simulink model "Simulink_Model_For_MAE_171a_Control_Lab"  (R2024b)
settings: Solver=VariableStepAuto  StartTime=0.0  StopTime=10.0  RelTol=1e-3
values from neighbouring files (symbols this model uses):
  den = [2.05e-15, 4.409e-13, 4.2e-12, 3.369e-10, 1.002e-09, 3.253e-08]    [Kasey_PID_tuner.m]    (also in kennyPIDtesting.m = [2.05e-15 4.409e-13 4.2e-12 3.369e-10 1.002e-09 3.253e-08])
  Kd = C.Kd    [Kasey_PID_tuner.m]    (also in kennyPIDtesting.m = 0.02)
  Ki = C.Ki    [Kasey_PID_tuner.m]    (also in kennyPIDtesting.m = 0.468)
  Kp = C.Kp    [Kasey_PID_tuner.m]    (also in kennyPIDtesting.m = 0.2)
  num = [6.04e-09, 1.088e-08, 1.434e-06]    [Kasey_PID_tuner.m]    (also in kennyPIDtesting.m = [6.04e-09 1.088e-08 1.434e-06])
settings Model: Creator=aidan  LastModifiedBy=aidan

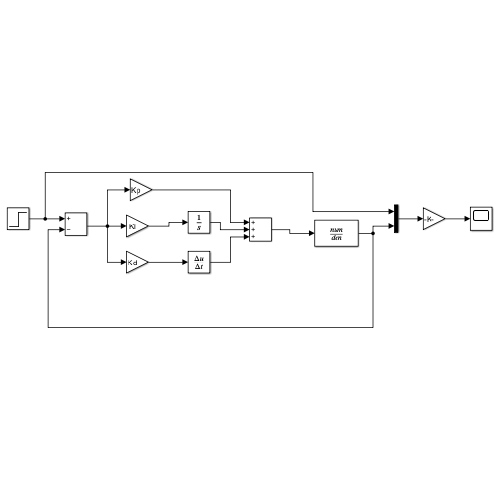
[thumbnail: Simulink's stored preview of the top-level diagram]
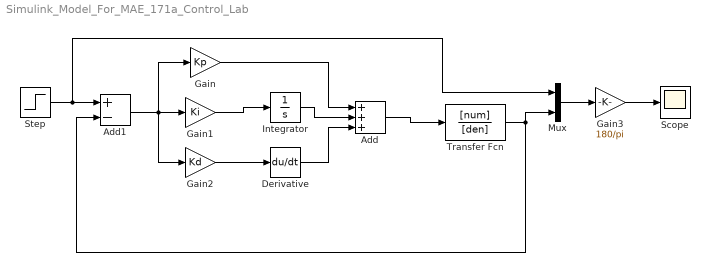
== system Simulink_Model_For_MAE_171a_Control_Lab ==
  Add : Sum  Inputs=+++
  Add1 : Sum  Inputs=+-
  Derivative : Derivative
  Gain : Gain  Gain=Kp
  Gain1 : Gain  Gain=Ki
  Gain2 : Gain  Gain=Kd
  Gain3 : Gain  Gain=180/pi
  Integrator : Integrator
  Mux : Mux  Inputs=2
  Scope : Scope
  Step : Step  SampleTime=0
  Transfer Fcn : TransferFcn  Numerator=[num]  Denominator=[den]
  wires:
  Gain2/1 -> Derivative/1
  Gain1/1 -> Integrator/1
  Gain/1 -> Add/1
  Integrator/1 -> Add/2
  Derivative/1 -> Add/3
  Add/1 -> Transfer Fcn/1
  Step/1 -> Mux/1, Add1/1
  Add1/1 -> Gain2/1, Gain1/1, Gain/1
  Transfer Fcn/1 -> Mux/2, Add1/2
  Mux/1 -> Gain3/1
  Gain3/1 -> Scope/1
